simulink model "APP_Model"  (R2024a)
settings: Solver=FixedStepDiscrete  StartTime=0.0  StopTime=1  RelTol=1e-3
libraries: simulink x2, pil_lib x1
settings Model: Creator=Bsmala  LastModifiedBy=Bsmala
settings OptimizationCC: DefaultParameterBehavior=Inlined  UseDivisionForNetSlopeComputation=on  GainParamInheritBuiltInType=on  UseFloatMulNetSlope=on  InlineInvariantSignals=on  PassReuseOutputArgsAs=Individual arguments  ZeroExternalMemoryAtStartup=off  ZeroInternalMemoryAtStartup=off  NoFixptDivByZeroProtection=on  EfficientFloat2IntCast=on  LifeSpan=1  OptimizeBlockOrder=speed  DifferentSizesBufferReuse=on  EfficientTunableParamExpr=on
settings DebuggingCC: ParameterTunabilityLossMsg=error  SFUnexpectedBacktrackingDiag=warning  SFNoUnconditionalDefaultTransitionDiag=warning
settings HardwareCC: ProdBitPerPointer=32  ProdBitPerSizeT=32  ProdBitPerPtrDiffT=32  ProdLargestAtomicInteger=Long  ProdLargestAtomicFloat=Double  ProdWordSize=32  ProdLongLongMode=on  ProdHWDeviceType=ARM Compatible->ARM Cortex-M
settings SFSimCC: MATLABDynamicMemAlloc=off
settings RTWCC: Description=Embedded Coder  SystemTargetFile=ert.tlc  TemplateMakefile=ert_default_tmf  GenerateReport=on  BuildConfiguration=Debug  LaunchReport=on
settings CodeAppCC: ForceParamTrailComments=on  IgnoreCustomStorageClasses=off  OperatorAnnotations=on  SimulinkDataObjDesc=on  SFDataObjDesc=on  CustomSymbolStrGlobalVar=rt$N$M  CustomSymbolStrType=$N$M  CustomSymbolStrFcn=$N$M$F  CustomSymbolStrMacro=$N$M  InsertBlockDesc=on  EnableCustomComments=on
settings ERTTargetCC: TargetLangStandard=C99 (ISO)  GenerateSampleERTMain=on  IncludeMdlTerminateFcn=off  CombineSignalStateStructs=on  SupportComplex=off  SupportContinuousTime=on  SupportNonInlinedSFcns=on  InlinedParameterPlacement=NonHierarchical  ERTCustomFileTemplate=example_file_process.tlc  ERTFilePackagingFormat=CompactWithDataFile

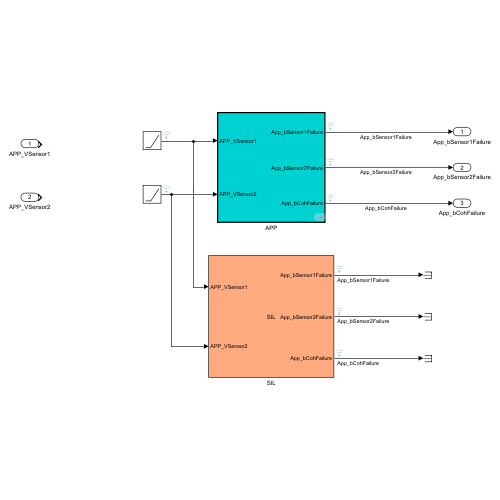
[thumbnail: Simulink's stored preview of the top-level diagram]
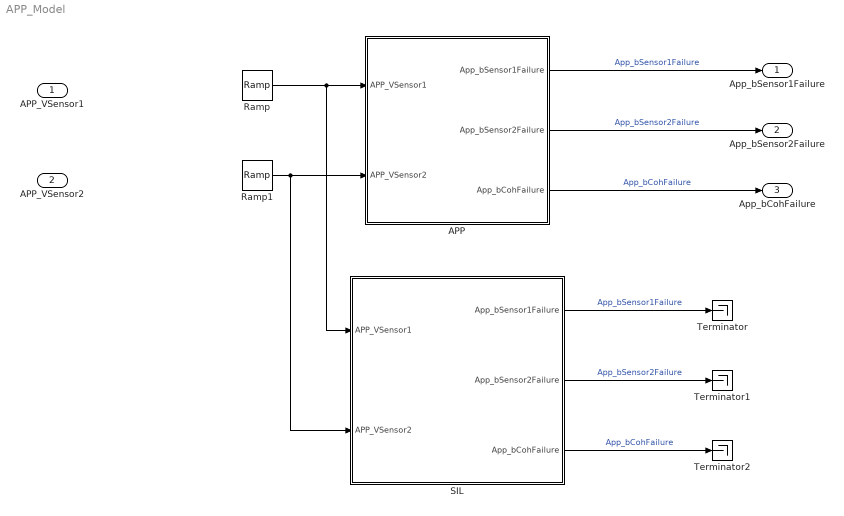
== system APP_Model ==
  APP_VSensor1 : Inport
  APP_VSensor2 : Inport  Port=2
  APP : Subsystem  TreatAsAtomicUnit=on
      settings: RTWSystemCode=Nonreusable function
  Ramp : simulink/Sources/Ramp  slope=4  start=0  InitialOutput=0.5
  Ramp1 : simulink/Sources/Ramp  slope=-4  start=0  InitialOutput=4.5
  SIL : Subsystem  Tag=__SL_testing_harness_stub_  DialogController=pil_create_dialog  LoadFcn=|
      | try
      |    if ~strcmp(rtw.pil.getPILVersion, '24.1 (R2024a)_15')
      |       set_param(gcb, 'DialogController', '');
      |       set_param(gcb, 'DialogControllerArgs', '');
      |    end
      | catch e
      |       set_param(gcb, 'DialogController', '');
      |       set_param(gcb, 'DialogControllerArgs', '');
      | end
      mask help: PIL:pil:XILBlockMaskDesc
      mask Display: disp('SIL');
  Terminator : Terminator
  Terminator1 : Terminator
  Terminator2 : Terminator
  App_bSensor1Failure : Outport
  App_bSensor2Failure : Outport  Port=2
  App_bCohFailure : Outport  Port=3
  wires:
  APP/1(App_bSensor1Failure) -> App_bSensor1Failure/1  "App_bSensor1Failure"
  APP/2(App_bSensor2Failure) -> App_bSensor2Failure/1  "App_bSensor2Failure"
  APP/3(App_bCohFailure) -> App_bCohFailure/1  "App_bCohFailure"
  Ramp/1 -> SIL/1(APP_VSensor1), APP/1(APP_VSensor1)
  Ramp1/1 -> SIL/2(APP_VSensor2), APP/2(APP_VSensor2)
  SIL/1(App_bSensor1Failure) -> Terminator/1  "App_bSensor1Failure"
  SIL/2(App_bSensor2Failure) -> Terminator1/1  "App_bSensor2Failure"
  SIL/3(App_bCohFailure) -> Terminator2/1  "App_bCohFailure"

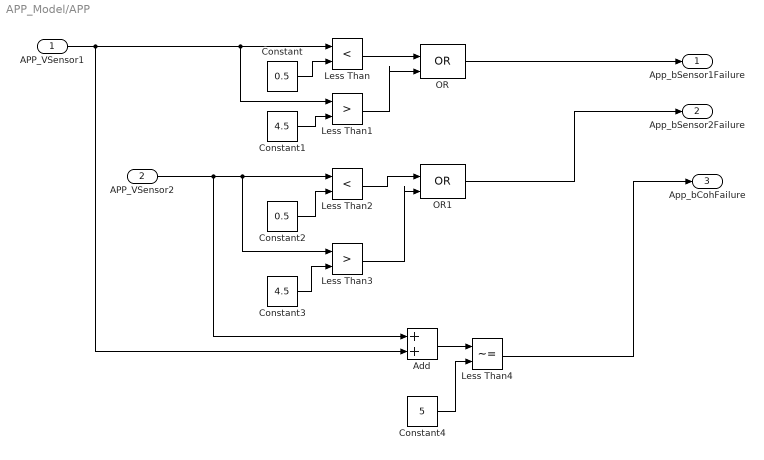
== system APP_Model/APP ==
  APP_VSensor1 : Inport
  APP_VSensor2 : Inport  Port=2
  Add : Sum
  Constant : Constant  Value=0.5
  Constant1 : Constant  Value=4.5
  Constant2 : Constant  Value=0.5
  Constant3 : Constant  Value=4.5
  Constant4 : Constant  Value=5
  Less Than : RelationalOperator  Operator=<  OutDataTypeStr=boolean  RndMeth=Simplest  InputSameDT=off
  Less Than1 : RelationalOperator  Operator=>  OutDataTypeStr=boolean  RndMeth=Simplest  InputSameDT=off
  Less Than2 : RelationalOperator  Operator=<  OutDataTypeStr=boolean  RndMeth=Simplest  InputSameDT=off
  Less Than3 : RelationalOperator  Operator=>  OutDataTypeStr=boolean  RndMeth=Simplest  InputSameDT=off
  Less Than4 : RelationalOperator  Operator=~=  OutDataTypeStr=boolean  RndMeth=Simplest  InputSameDT=off
  OR : Logic  Operator=OR  IconShape=distinctive  AllPortsSameDT=off  OutDataTypeStr=boolean
  OR1 : Logic  Operator=OR  IconShape=distinctive  AllPortsSameDT=off  OutDataTypeStr=boolean
  App_bSensor1Failure : Outport
  App_bSensor2Failure : Outport  Port=2
  App_bCohFailure : Outport  Port=3
  wires:
  Less Than4/1 -> App_bCohFailure/1
  APP_VSensor1/1 -> Less Than1/1, Less Than/1, Add/2
  APP_VSensor2/1 -> Add/1, Less Than3/1, Less Than2/1
  Constant/1 -> Less Than/2
  Constant3/1 -> Less Than3/2
  Constant1/1 -> Less Than1/2
  Constant2/1 -> Less Than2/2
  Less Than/1 -> OR/1
  Less Than3/1 -> OR1/2
  Add/1 -> Less Than4/1
  Less Than2/1 -> OR1/1
  Less Than1/1 -> OR/2
  Constant4/1 -> Less Than4/2
  OR/1 -> App_bSensor1Failure/1
  OR1/1 -> App_bSensor2Failure/1

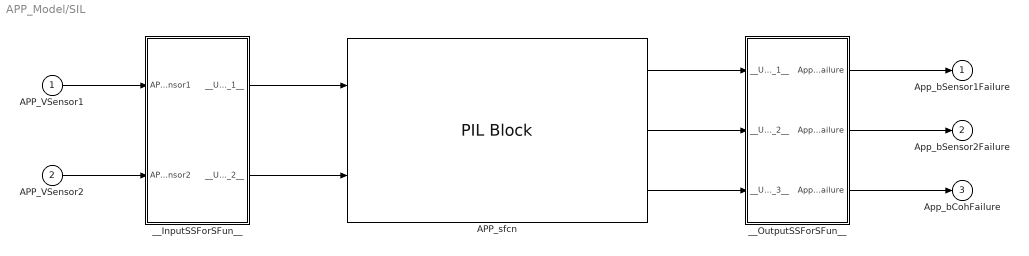
== system APP_Model/SIL ==
  APP_VSensor1 : Inport
  APP_VSensor2 : Inport  Port=2
  APP_sfcn : pil_lib/PIL Block  SimulationMode=SIL  IsTopModelPIL=off  CodeDir=APP0_ert_rtw  AnchorDir=C:\bsmala\MBD  ConfigName=Software-in-the-Loop (SIL)  XrelIsTopModelCode=on  XrelIsReusable=off  XrelDWorkNames={}  XrelDWorkTypes={}  XrelModelArgVals={}  XrelOrderedParamNames={}  XRelNonFiniteStyle=NONFINITE_UNUSED
  __InputSSForSFun__ : Subsystem
  __OutputSSForSFun__ : Subsystem
  App_bSensor1Failure : Outport
  App_bSensor2Failure : Outport  Port=2
  App_bCohFailure : Outport  Port=3
  wires:
  __OutputSSForSFun__/3(App_bCohFailure) -> App_bCohFailure/1
  __OutputSSForSFun__/2(App_bSensor2Failure) -> App_bSensor2Failure/1
  __OutputSSForSFun__/1(App_bSensor1Failure) -> App_bSensor1Failure/1
  APP_sfcn/3 -> __OutputSSForSFun__/3(__UniqueInportName__3__)
  APP_sfcn/2 -> __OutputSSForSFun__/2(__UniqueInportName__2__)
  APP_sfcn/1 -> __OutputSSForSFun__/1(__UniqueInportName__1__)
  __InputSSForSFun__/2(__UniqueOutportName__2__) -> APP_sfcn/2
  __InputSSForSFun__/1(__UniqueOutportName__1__) -> APP_sfcn/1
  APP_VSensor2/1 -> __InputSSForSFun__/2(APP_VSensor2)
  APP_VSensor1/1 -> __InputSSForSFun__/1(APP_VSensor1)

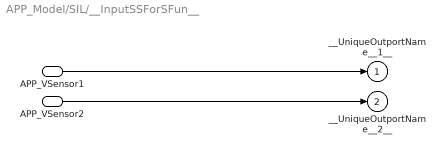
== system APP_Model/SIL/__InputSSForSFun__ ==
  APP_VSensor1 : Inport
  APP_VSensor2 : Inport  Port=2
  __UniqueOutportName__1__ : Outport
  __UniqueOutportName__2__ : Outport  Port=2
  wires:
  APP_VSensor2/1 -> __UniqueOutportName__2__/1
  APP_VSensor1/1 -> __UniqueOutportName__1__/1

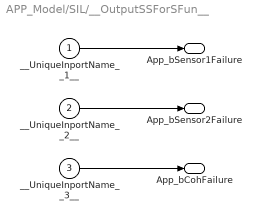
== system APP_Model/SIL/__OutputSSForSFun__ ==
  __UniqueInportName__1__ : Inport
  __UniqueInportName__2__ : Inport  Port=2
  __UniqueInportName__3__ : Inport  Port=3
  App_bSensor1Failure : Outport
  App_bSensor2Failure : Outport  Port=2
  App_bCohFailure : Outport  Port=3
  wires:
  __UniqueInportName__3__/1 -> App_bCohFailure/1
  __UniqueInportName__2__/1 -> App_bSensor2Failure/1
  __UniqueInportName__1__/1 -> App_bSensor1Failure/1
